simulink model "RaibertControlV10"  (R2022a)
settings: Solver=ode23t  StartTime=0.0  StopTime=10  FixedStep=1/1000  MaxStep=0.001  RelTol=1e-3  AbsTol=1e-3  EnableMultiTasking=on
values from neighbouring files (symbols this model uses):
  dphi_d_14 = 0.0    (= 0)    [initialization.m]
  dphi_d_23 = 0.0    (= 0)    [initialization.m]
  dphi_des = DesiredImpedenceValues(4)    [Controller.m]    (also in initialization.m = 0)
  dr_d_14 = 0.0    (= 0)    [initialization.m]
  dr_d_23 = 0.0    (= 0)    [initialization.m]
  dr_des = DesiredImpedenceValues(3)    [Controller.m]    (also in initialization.m = 0)
  Fpush_d_14 = 300    [initialization.m]
  Fpush_d_23 = 300    [initialization.m]
  GAIN_dx_d_14 = 0.05    [initialization.m]
  GAIN_dx_d_23 = 0.05    [initialization.m]
  Kd_phi_d_14 = 10    [initialization.m]
  Kd_phi_d_23 = 10    [initialization.m]
  Kd_r_d_14 = Kp_r_d_14*0.1    (= 60)    [initialization.m]
  Kd_r_d_23 = Kp_r_d_23*0.1    (= 50)    [initialization.m]
  Kdphi_des = DesiredImpedenceValues(8)    [Controller.m]    (also in initialization.m = 5)
  Kdr_des = DesiredImpedenceValues(6)    [Controller.m]    (also in initialization.m = 700)
  Kp_phi_d_14 = 200    [initialization.m]
  Kp_phi_d_23 = 200    [initialization.m]
  Kp_r_d_14 = 600    [initialization.m]
  Kp_r_d_23 = 500    [initialization.m]
  Kpphi_des = DesiredImpedenceValues(7)    [Controller.m]    (also in initialization.m = 50)
  Kpr_des = DesiredImpedenceValues(5)    [Controller.m]    (also in initialization.m = 700)
  phi_d_14 = 0    [initialization.m]
  phi_d_23 = 0    [initialization.m]
  phi_des = DesiredImpedenceValues(2)    [Controller.m]    (also in initialization.m = 0)
  r_d_14 = 0.38    [initialization.m]
  r_d_23 = 0.38    [initialization.m]
  r_des = DesiredImpedenceValues(1)    [Controller.m]    (also in initialization.m = 0.4)
  rthrust_d_14 = 0.3    [initialization.m]
  rthrust_d_23 = 0.3    [initialization.m]
undefined symbols (not defined in the file or in its folder): Carrier, N, Ring, T, X, Y, Z
libraries: sm_lib x136, nesl_utility x25, Multibody_Parts_Lib x4, fl_lib x4
(part 7 of 8)

== matlab function RaibertControlV10/Raibert Control14/to_dPolar ==
  data: M1_State input; dr output; dphi output; M4_State input
function [dr,dphi] = Velocity(M1_State,M4_State)
%VELOCITY
%    [DR,DPHI] = VELOCITY(THETA1,THETA2,DTHETA1,DTHETA2)

%    This function was generated by the Symbolic Math Toolbox version 8.6.
%    17-May-2022 09:32:08
theta1 = M4_State.q;
dtheta1 = M4_State.w;
theta2 = M1_State.q;
dtheta2 = M1_State.w;
dr = dtheta1.*(sin(acos(sqrt((sin(theta1-pi./2.0).*(7.0./4.0e+1)+sin(theta2+pi./2.0).*(7.0./4.0e+1)).^2+abs(cos(theta1-pi./2.0).*(7.0./4.0e+1)+cos(theta2+pi./2.0).*(7.0./4.0e+1)+3.0./2.5e+1).^2).*(5.0./3.0))+atan2(sin(theta1-pi./2.0).*(-7.0./4.0e+1)-sin(theta2+pi./2.0).*(7.0./4.0e+1),abs(cos(theta1-pi./2.0).*(7.0./4.0e+1)+cos(theta2+pi./2.0).*(7.0./4.0e+1)+3.0./2.5e+1))+6.012387278395987e-2).*(1.0./sqrt((sin(theta1-pi./2.0).*(7.0./4.0e+1)+sin(theta2+pi./2.0).*(7.0./4.0e+1)).^2+abs(cos(theta1-pi./2.0).*(7.0./4.0e+1)+cos(theta2+pi./2.0).*(7.0./4.0e+1)+3.0./2.5e+1).^2).*(cos(theta1-pi./2.0).*(sin(theta1-pi./2.0).*(7.0./4.0e+1)+sin(theta2+pi./2.0).*(7.0./4.0e+1)).*(7.0./2.0e+1)-abs(cos(theta1-pi./2.0).*(7.0./4.0e+1)+cos(theta2+pi./2.0).*(7.0./4.0e+1)+3.0./2.5e+1).*sign(cos(theta1-pi./2.0).*(7.0./4.0e+1)+cos(theta2+pi./2.0).*(7.0./4.0e+1)+3.0./2.5e+1).*sin(theta1-pi./2.0).*(7.0./2.0e+1)).*1.0./sqrt((sin(theta1-pi./2.0).*(7.0./4.0e+1)+sin(theta2+pi./2.0).*(7.0./4.0e+1)).^2.*(-2.5e+1./9.0)-abs(cos(theta1-pi./2.0).*(7.0./4.0e+1)+cos(theta2+pi./2.0).*(7.0./4.0e+1)+3.0./2.5e+1).^2.*(2.5e+1./9.0)+1.0).*(5.0./6.0)+(abs(cos(theta1-pi./2.0).*(7.0./4.0e+1)+cos(theta2+pi./2.0).*(7.0./4.0e+1)+3.0./2.5e+1).^2.*((cos(theta1-pi./2.0).*(7.0./4.0e+1))./abs(cos(theta1-pi./2.0).*(7.0./4.0e+1)+cos(theta2+pi./2.0).*(7.0./4.0e+1)+3.0./2.5e+1)+1.0./abs(cos(theta1-pi./2.0).*(7.0./4.0e+1)+cos(theta2+pi./2.0).*(7.0./4.0e+1)+3.0./2.5e+1).^2.*sign(cos(theta1-pi./2.0).*(7.0./4.0e+1)+cos(theta2+pi./2.0).*(7.0./4.0e+1)+3.0./2.5e+1).*sin(theta1-pi./2.0).*(sin(theta1-pi./2.0).*(7.0./4.0e+1)+sin(theta2+pi./2.0).*(7.0./4.0e+1)).*(7.0./4.0e+1)))./((sin(theta1-pi./2.0).*(7.0./4.0e+1)+sin(theta2+pi./2.0).*(7.0./4.0e+1)).^2+abs(cos(theta1-pi./2.0).*(7.0./4.0e+1)+cos(theta2+pi./2.0).*(7.0./4.0e+1)+3.0./2.5e+1).^2)).*(cos(acos(sqrt((sin(theta1-pi./2.0).*(7.0./4.0e+1)+sin(theta2+pi./2.0).*(7.0./4.0e+1)).^2+abs(cos(theta1-pi./2.0).*(7.0./4.0e+1)+cos(theta2+pi./2.0).*(7.0./4.0e+1)+3.0./2.5e+1).^2).*(5.0./3.0))+atan2(sin(theta1-pi./2.0).*(-7.0./4.0e+1)-sin(theta2+pi./2.0).*(7.0./4.0e+1),abs(cos(theta1-pi./2.0).*(7.0./4.0e+1)+cos(theta2+pi./2.0).*(7.0./4.0e+1)+3.0./2.5e+1))+6.012387278395987e-2).*(-3.328470665197855e-1)+cos(theta2+pi./2.0).*(7.0./4.0e+1)+3.0./5.0e+1).*6.65694133039571e-1+cos(acos(sqrt((sin(theta1-pi./2.0).*(7.0./4.0e+1)+sin(theta2+pi./2.0).*(7.0./4.0e+1)).^2+abs(cos(theta1-pi./2.0).*(7.0./4.0e+1)+cos(theta2+pi./2.0).*(7.0./4.0e+1)+3.0./2.5e+1).^2).*(5.0./3.0))+atan2(sin(theta1-pi./2.0).*(-7.0./4.0e+1)-sin(theta2+pi./2.0).*(7.0./4.0e+1),abs(cos(theta1-pi./2.0).*(7.0./4.0e+1)+cos(theta2+pi./2.0).*(7.0./4.0e+1)+3.0./2.5e+1))+6.012387278395987e-2).*(sin(acos(sqrt((sin(theta1-pi./2.0).*(7.0./4.0e+1)+sin(theta2+pi./2.0).*(7.0./4.0e+1)).^2+abs(cos(theta1-pi./2.0).*(7.0./4.0e+1)+cos(theta2+pi./2.0).*(7.0./4.0e+1)+3.0./2.5e+1).^2).*(5.0./3.0))+atan2(sin(theta1-pi./2.0).*(-7.0./4.0e+1)-sin(theta2+pi./2.0).*(7.0./4.0e+1),abs(cos(theta1-pi./2.0).*(7.0./4.0e+1)+cos(theta2+pi./2.0).*(7.0./4.0e+1)+3.0./2.5e+1))+6.012387278395987e-2).*3.328470665197855e-1+sin(theta2+pi./2.0).*(7.0./4.0e+1)).*(1.0./sqrt((sin(theta1-pi./2.0).*(7.0./4.0e+1)+sin(theta2+pi./2.0).*(7.0./4.0e+1)).^2+abs(cos(theta1-pi./2.0).*(7.0./4.0e+1)+cos(theta2+pi./2.0).*(7.0./4.0e+1)+3.0./2.5e+1).^2).*(cos(theta1-pi./2.0).*(sin(theta1-pi./2.0).*(7.0./4.0e+1)+sin(theta2+pi./2.0).*(7.0./4.0e+1)).*(7.0./2.0e+1)-abs(cos(theta1-pi./2.0).*(7.0./4.0e+1)+cos(theta2+pi./2.0).*(7.0./4.0e+1)+3.0./2.5e+1).*sign(cos(theta1-pi./2.0).*(7.0./4.0e+1)+cos(theta2+pi./2.0).*(7.0./4.0e+1)+3.0./2.5e+1).*sin(theta1-pi./2.0).*(7.0./2.0e+1)).*1.0./sqrt((sin(theta1-pi./2.0).*(7.0./4.0e+1)+sin(theta2+pi./2.0).*(7.0./4.0e+1)).^2.*(-2.5e+1./9.0)-abs(cos(theta1-pi./2.0).*(7.0./4.0e+1)+cos(theta2+pi./2.0).*(7.0./4.0e+1)+3.0./2.5e+1).^2.*(2.5e+1./9.0)+1.0).*(5.0./6.0)+(abs(cos(theta1-pi./2.0).*(7.0./4.0e+1)+cos(theta2+pi./2.0).*(7.0./4.0e+1)+3.0./2.5e+1).^2.*((cos(theta1-pi./2.0).*(7.0./4.0e+1))./abs(cos(theta1-pi./2.0).*(7.0./4.0e+1)+cos(theta2+pi./2.0).*(7.0./4.0e+1)+3.0./2.5e+1)+1.0./abs(cos(theta1-pi./2.0).*(7.0./4.0e+1)+cos(theta2+pi./2.0).*(7.0./4.0e+1)+3.0./2.5e+1).^2.*sign(cos(theta1-pi./2.0).*(7.0./4.0e+1)+cos(theta2+pi./2.0).*(7.0./4.0e+1)+3.0./2.5e+1).*sin(theta1-pi./2.0).*(sin(theta1-pi./2.0).*(7.0./4.0e+1)+sin(theta2+pi./2.0).*(7.0./4.0e+1)).*(7.0./4.0e+1)))./((sin(theta1-pi./2.0).*(7.0./4.0e+1)+sin(theta2+pi./2.0).*(7.0./4.0e+1)).^2+abs(cos(theta1-pi./2.0).*(7.0./4.0e+1)+cos(theta2+pi./2.0).*(7.0./4.0e+1)+3.0./2.5e+1).^2)).*6.65694133039571e-1).*1.0./sqrt((cos(acos(sqrt((sin(theta1-pi./2.0).*(7.0./4.0e+1)+sin(theta2+pi./2.0).*(7.0./4.0e+1)).^2+abs(cos(theta1-pi./2.0).*(7.0./4.0e+1)+cos(theta2+pi./2.0).*(7.0./4.0e+1)+3.0./2.5e+1).^2).*(5.0./3.0))+atan2(sin(theta1-pi./2.0).*(-7.0./4.0e+1)-sin(theta2+pi./2.0).*(7.0./4.0e+1),abs(cos(theta1-pi./2.0).*(7.0./4.0e+1)+cos(theta2+pi./2.0).*(7.0./4.0e+1)+3.0./2.5e+1))+6.012387278395987e-2).*(-3.328470665197855e-1)+cos(theta2+pi./2.0).*(7.0./4.0e+1)+3.0./5.0e+1).^2+(sin(acos(sqrt((sin(theta1-pi./2.0).*(7.0./4.0e+1)+sin(theta2+pi./2.0).*(7.0./4.0e+1)).^2+abs(cos(theta1-pi./2.0).*(7.0./4.0e+1)+cos(theta2+pi./2.0).*(7.0./4.0e+1)+3.0./2.5e+1).^2).*(5.0./3.0))+atan2(sin(theta1-pi./2.0).*(-7.0./4.0e+1)-sin(theta2+pi./2.0).*(7.0./4.0e+1),abs(cos(theta1-pi./2.0).*(7.0./4.0e+1)+cos(theta2+pi./2.0).*(7.0./4.0e+1)+3.0./2.5e+1))+6.012387278395987e-2).*3.328470665197855e-1+sin(theta2+pi./2.0).*(7.0./4.0e+1)).^2).*(-1.0./2.0)+(dtheta2.*((sin(acos(sqrt((sin(theta1-pi./2.0).*(7.0./4.0e+1)+sin(theta2+pi./2.0).*(7.0./4.0e+1)).^2+abs(cos(theta1-pi./2.0).*(7.0./4.0e+1)+cos(theta2+pi./2.0).*(7.0./4.0e+1)+3.0./2.5e+1).^2).*(5.0./3.0))+atan2(sin(theta1-pi./2.0).*(-7.0./4.0e+1)-sin(theta2+pi./2.0).*(7.0./4.0e+1),abs(cos(theta1-pi./2.0).*(7.0./4.0e+1)+cos(theta2+pi./2.0).*(7.0./4.0e+1)+3.0./2.5e+1))+6.012387278395987e-2).*3.328470665197855e-1+sin(theta2+pi./2.0).*(7.0./4.0e+1)).*(cos(theta2+pi./2.0).*(7.0./4.0e+1)-cos(acos(sqrt((sin(theta1-pi./2.0).*(7.0./4.0e+1)+sin(theta2+pi./2.0).*(7.0./4.0e+1)).^2+abs(cos(theta1-pi./2.0).*(7.0./4.0e+1)+cos(theta2+pi./2.0).*(7.0./4.0e+1)+3.0./2.5e+1).^2).*(5.0./3.0))+atan2(sin(theta1-pi./2.0).*(-7.0./4.0e+1)-sin(theta2+pi./2.0).*(7.0./4.0e+1),abs(cos(theta1-pi./2.0).*(7.0./4.0e+1)+cos(theta2+pi./2.0).*(7.0./4.0e+1)+3.0./2.5e+1))+6.012387278395987e-2).*(1.0./sqrt((sin(theta1-pi./2.0).*(7.0./4.0e+1)+sin(theta2+pi./2.0).*(7.0./4.0e+1)).^2+abs(cos(theta1-pi./2.0).*(7.0./4.0e+1)+cos(theta2+pi./2.0).*(7.0./4.0e+1)+3.0./2.5e+1).^2).*(cos(theta2+pi./2.0).*(sin(theta1-pi./2.0).*(7.0./4.0e+1)+sin(theta2+pi./2.0).*(7.0./4.0e+1)).*(7.0./2.0e+1)-abs(cos(theta1-pi./2.0).*(7.0./4.0e+1)+cos(theta2+pi./2.0).*(7.0./4.0e+1)+3.0./2.5e+1).*sign(cos(theta1-pi./2.0).*(7.0./4.0e+1)+cos(theta2+pi./2.0).*(7.0./4.0e+1)+3.0./2.5e+1).*sin(theta2+pi./2.0).*(7.0./2.0e+1)).*1.0./sqrt((sin(theta1-pi./2.0).*(7.0./4.0e+1)+sin(theta2+pi./2.0).*(7.0./4.0e+1)).^2.*(-2.5e+1./9.0)-abs(cos(theta1-pi./2.0).*(7.0./4.0e+1)+cos(theta2+pi./2.0).*(7.0./4.0e+1)+3.0./2.5e+1).^2.*(2.5e+1./9.0)+1.0).*(5.0./6.0)+(abs(cos(theta1-pi./2.0).*(7.0./4.0e+1)+cos(theta2+pi./2.0).*(7.0./4.0e+1)+3.0./2.5e+1).^2.*((cos(theta2+pi./2.0).*(7.0./4.0e+1))./abs(cos(theta1-pi./2.0).*(7.0./4.0e+1)+cos(theta2+pi./2.0).*(7.0./4.0e+1)+3.0./2.5e+1)+1.0./abs(cos(theta1-pi./2.0).*(7.0./4.0e+1)+cos(theta2+pi./2.0).*(7.0./4.0e+1)+3.0./2.5e+1).^2.*sign(cos(theta1-pi./2.0).*(7.0./4.0e+1)+cos(theta2+pi./2.0).*(7.0./4.0e+1)+3.0./2.5e+1).*sin(theta2+pi./2.0).*(sin(theta1-pi./2.0).*(7.0./4.0e+1)+sin(theta2+pi./2.0).*(7.0./4.0e+1)).*(7.0./4.0e+1)))./((sin(theta1-pi./2.0).*(7.0./4.0e+1)+sin(theta2+pi./2.0).*(7.0./4.0e+1)).^2+abs(cos(theta1-pi./2.0).*(7.0./4.0e+1)+cos(theta2+pi./2.0).*(7.0./4.0e+1)+3.0./2.5e+1).^2)).*3.328470665197855e-1).*2.0-(sin(theta2+pi./2.0).*(7.0./4.0e+1)+sin(acos(sqrt((sin(theta1-pi./2.0).*(7.0./4.0e+1)+sin(theta2+pi./2.0).*(7.0./4.0e+1)).^2+abs(cos(theta1-pi./2.0).*(7.0./4.0e+1)+cos(theta2+pi./2.0).*(7.0./4.0e+1)+3.0./2.5e+1).^2).*(5.0./3.0))+atan2(sin(theta1-pi./2.0).*(-7.0./4.0e+1)-sin(theta2+pi./2.0).*(7.0./4.0e+1),abs(cos(theta1-pi./2.0).*(7.0./4.0e+1)+cos(theta2+pi./2.0).*(7.0./4.0e+1)+3.0./2.5e+1))+6.012387278395987e-2).*(1.0./sqrt((sin(theta1-pi./2.0).*(7.0./4.0e+1)+sin(theta2+pi./2.0).*(7.0./4.0e+1)).^2+abs(cos(theta1-pi./2.0).*(7.0./4.0e+1)+cos(theta2+pi./2.0).*(7.0./4.0e+1)+3.0./2.5e+1).^2).*(cos(theta2+pi./2.0).*(sin(theta1-pi./2.0).*(7.0./4.0e+1)+sin(theta2+pi./2.0).*(7.0./4.0e+1)).*(7.0./2.0e+1)-abs(cos(theta1-pi./2.0).*(7.0./4.0e+1)+cos(theta2+pi./2.0).*(7.0./4.0e+1)+3.0./2.5e+1).*sign(cos(theta1-pi./2.0).*(7.0./4.0e+1)+cos(theta2+pi./2.0).*(7.0./4.0e+1)+3.0./2.5e+1).*sin(theta2+pi./2.0).*(7.0./2.0e+1)).*1.0./sqrt((sin(theta1-pi./2.0).*(7.0./4.0e+1)+sin(theta2+pi./2.0).*(7.0./4.0e+1)).^2.*(-2.5e+1./9.0)-abs(cos(theta1-pi./2.0).*(7.0./4.0e+1)+cos(theta2+pi./2.0).*(7.0./4.0e+1)+3.0./2.5e+1).^2.*(2.5e+1./9.0)+1.0).*(5.0./6.0)+(abs(cos(theta1-pi./2.0).*(7.0./4.0e+1)+cos(theta2+pi./2.0).*(7.0./4.0e+1)+3.0./2.5e+1).^2.*((cos(theta2+pi./2.0).*(7.0./4.0e+1))./abs(cos(theta1-pi./2.0).*(7.0./4.0e+1)+cos(theta2+pi./2.0).*(7.0./4.0e+1)+3.0./2.5e+1)+1.0./abs(cos(theta1-pi./2.0).*(7.0./4.0e+1)+cos(theta2+pi./2.0).*(7.0./4.0e+1)+3.0./2.5e+1).^2.*sign(cos(theta1-pi./2.0).*(7.0./4.0e+1)+cos(theta2+pi./2.0).*(7.0./4.0e+1)+3.0./2.5e+1).*sin(theta2+pi./2.0).*(sin(theta1-pi./2.0).*(7.0./4.0e+1)+sin(theta2+pi./2.0).*(7.0./4.0e+1)).*(7.0./4.0e+1)))./((sin(theta1-pi./2.0).*(7.0./4.0e+1)+sin(theta2+pi./2.0).*(7.0./4.0e+1)).^2+abs(cos(theta1-pi./2.0).*(7.0./4.0e+1)+cos(theta2+pi./2.0).*(7.0./4.0e+1)+3.0./2.5e+1).^2)).*3.328470665197855e-1).*(cos(acos(sqrt((sin(theta1-pi./2.0).*(7.0./4.0e+1)+sin(theta2+pi./2.0).*(7.0./4.0e+1)).^2+abs(cos(theta1-pi./2.0).*(7.0./4.0e+1)+cos(theta2+pi./2.0).*(7.0./4.0e+1)+3.0./2.5e+1).^2).*(5.0./3.0))+atan2(sin(theta1-pi./2.0).*(-7.0./4.0e+1)-sin(theta2+pi./2.0).*(7.0./4.0e+1),abs(cos(theta1-pi./2.0).*(7.0./4.0e+1)+cos(theta2+pi./2.0).*(7.0./4.0e+1)+3.0./2.5e+1))+6.012387278395987e-2).*(-3.328470665197855e-1)+cos(theta2+pi./2.0).*(7.0./4.0e+1)+3.0./5.0e+1).*2.0).*1.0./sqrt((cos(acos(sqrt((sin(theta1-pi./2.0).*(7.0./4.0e+1)+sin(theta2+pi./2.0).*(7.0./4.0e+1)).^2+abs(cos(theta1-pi./2.0).*(7.0./4.0e+1)+cos(theta2+pi./2.0).*(7.0./4.0e+1)+3.0./2.5e+1).^2).*(5.0./3.0))+atan2(sin(theta1-pi./2.0).*(-7.0./4.0e+1)-sin(theta2+pi./2.0).*(7.0./4.0e+1),abs(cos(theta1-pi./2.0).*(7.0./4.0e+1)+cos(theta2+pi./2.0).*(7.0./4.0e+1)+3.0./2.5e+1))+6.012387278395987e-2).*(-3.328470665197855e-1)+cos(theta2+pi./2.0).*(7.0./4.0e+1)+3.0./5.0e+1).^2+(sin(acos(sqrt((sin(theta1-pi./2.0).*(7.0./4.0e+1)+sin(theta2+pi./2.0).*(7.0./4.0e+1)).^2+abs(cos(theta1-pi./2.0).*(7.0./4.0e+1)+cos(theta2+pi./2.0).*(7.0./4.0e+1)+3.0./2.5e+1).^2).*(5.0./3.0))+atan2(sin(theta1-pi./2.0).*(-7.0./4.0e+1)-sin(theta2+pi./2.0).*(7.0./4.0e+1),abs(cos(theta1-pi./2.0).*(7.0./4.0e+1)+cos(theta2+pi./2.0).*(7.0./4.0e+1)+3.0./2.5e+1))+6.012387278395987e-2).*3.328470665197855e-1+sin(theta2+pi./2.0).*(7.0./4.0e+1)).^2))./2.0;
if nargout > 1
    dphi = (dtheta1.*((cos(acos(sqrt((sin(theta1-pi./2.0).*(7.0./4.0e+1)+sin(theta2+pi./2.0).*(7.0./4.0e+1)).^2+abs(cos(theta1-pi./2.0).*(7.0./4.0e+1)+cos(theta2+pi./2.0).*(7.0./4.0e+1)+3.0./2.5e+1).^2).*(5.0./3.0))+atan2(sin(theta1-pi./2.0).*(-7.0./4.0e+1)-sin(theta2+pi./2.0).*(7.0./4.0e+1),abs(cos(theta1-pi./2.0).*(7.0./4.0e+1)+cos(theta2+pi./2.0).*(7.0./4.0e+1)+3.0./2.5e+1))+6.012387278395987e-2).*(1.0./sqrt((sin(theta1-pi./2.0).*(7.0./4.0e+1)+sin(theta2+pi./2.0).*(7.0./4.0e+1)).^2+abs(cos(theta1-pi./2.0).*(7.0./4.0e+1)+cos(theta2+pi./2.0).*(7.0./4.0e+1)+3.0./2.5e+1).^2).*(cos(theta1-pi./2.0).*(sin(theta1-pi./2.0).*(7.0./4.0e+1)+sin(theta2+pi./2.0).*(7.0./4.0e+1)).*(7.0./2.0e+1)-abs(cos(theta1-pi./2.0).*(7.0./4.0e+1)+cos(theta2+pi./2.0).*(7.0./4.0e+1)+3.0./2.5e+1).*sign(cos(theta1-pi./2.0).*(7.0./4.0e+1)+cos(theta2+pi./2.0).*(7.0./4.0e+1)+3.0./2.5e+1).*sin(theta1-pi./2.0).*(7.0./2.0e+1)).*1.0./sqrt((sin(theta1-pi./2.0).*(7.0./4.0e+1)+sin(theta2+pi./2.0).*(7.0./4.0e+1)).^2.*(-2.5e+1./9.0)-abs(cos(theta1-pi./2.0).*(7.0./4.0e+1)+cos(theta2+pi./2.0).*(7.0./4.0e+1)+3.0./2.5e+1).^2.*(2.5e+1./9.0)+1.0).*(5.0./6.0)+(abs(cos(theta1-pi./2.0).*(7.0./4.0e+1)+cos(theta2+pi./2.0).*(7.0./4.0e+1)+3.0./2.5e+1).^2.*((cos(theta1-pi./2.0).*(7.0./4.0e+1))./abs(cos(theta1-pi./2.0).*(7.0./4.0e+1)+cos(theta2+pi./2.0).*(7.0./4.0e+1)+3.0./2.5e+1)+1.0./abs(cos(theta1-pi./2.0).*(7.0./4.0e+1)+cos(theta2+pi./2.0).*(7.0./4.0e+1)+3.0./2.5e+1).^2.*sign(cos(theta1-pi./2.0).*(7.0./4.0e+1)+cos(theta2+pi./2.0).*(7.0./4.0e+1)+3.0./2.5e+1).*sin(theta1-pi./2.0).*(sin(theta1-pi./2.0).*(7.0./4.0e+1)+sin(theta2+pi./2.0).*(7.0./4.0e+1)).*(7.0./4.0e+1)))./((sin(theta1-pi./2.0).*(7.0./4.0e+1)+sin(theta2+pi./2.0).*(7.0./4.0e+1)).^2+abs(cos(theta1-pi./2.0).*(7.0./4.0e+1)+cos(theta2+pi./2.0).*(7.0./4.0e+1)+3.0./2.5e+1).^2)).*3.328470665197855e-1)./(cos(acos(sqrt((sin(theta1-pi./2.0).*(7.0./4.0e+1)+sin(theta2+pi./2.0).*(7.0./4.0e+1)).^2+abs(cos(theta1-pi./2.0).*(7.0./4.0e+1)+cos(theta2+pi./2.0).*(7.0./4.0e+1)+3.0./2.5e+1).^2).*(5.0./3.0))+atan2(sin(theta1-pi./2.0).*(-7.0./4.0e+1)-sin(theta2+pi./2.0).*(7.0./4.0e+1),abs(cos(theta1-pi./2.0).*(7.0./4.0e+1)+cos(theta2+pi./2.0).*(7.0./4.0e+1)+3.0./2.5e+1))+6.012387278395987e-2).*(-3.328470665197855e-1)+cos(theta2+pi./2.0).*(7.0./4.0e+1)+3.0./5.0e+1)-sin(acos(sqrt((sin(theta1-pi./2.0).*(7.0./4.0e+1)+sin(theta2+pi./2.0).*(7.0./4.0e+1)).^2+abs(cos(theta1-pi./2.0).*(7.0./4.0e+1)+cos(theta2+pi./2.0).*(7.0./4.0e+1)+3.0./2.5e+1).^2).*(5.0./3.0))+atan2(sin(theta1-pi./2.0).*(-7.0./4.0e+1)-sin(theta2+pi./2.0).*(7.0./4.0e+1),abs(cos(theta1-pi./2.0).*(7.0./4.0e+1)+cos(theta2+pi./2.0).*(7.0./4.0e+1)+3.0./2.5e+1))+6.012387278395987e-2).*(sin(acos(sqrt((sin(theta1-pi./2.0).*(7.0./4.0e+1)+sin(theta2+pi./2.0).*(7.0./4.0e+1)).^2+abs(cos(theta1-pi./2.0).*(7.0./4.0e+1)+cos(theta2+pi./2.0).*(7.0./4.0e+1)+3.0./2.5e+1).^2).*(5.0./3.0))+atan2(sin(theta1-pi./2.0).*(-7.0./4.0e+1)-sin(theta2+pi./2.0).*(7.0./4.0e+1),abs(cos(theta1-pi./2.0).*(7.0./4.0e+1)+cos(theta2+pi./2.0).*(7.0./4.0e+1)+3.0./2.5e+1))+6.012387278395987e-2).*3.328470665197855e-1+sin(theta2+pi./2.0).*(7.0./4.0e+1)).*(1.0./sqrt((sin(theta1-pi./2.0).*(7.0./4.0e+1)+sin(theta2+pi./2.0).*(7.0./4.0e+1)).^2+abs(cos(theta1-pi./2.0).*(7.0./4.0e+1)+cos(theta2+pi./2.0).*(7.0./4.0e+1)+3.0./2.5e+1).^2).*(cos(theta1-pi./2.0).*(sin(theta1-pi./2.0).*(7.0./4.0e+1)+sin(theta2+pi./2.0).*(7.0./4.0e+1)).*(7.0./2.0e+1)-abs(cos(theta1-pi./2.0).*(7.0./4.0e+1)+cos(theta2+pi./2.0).*(7.0./4.0e+1)+3.0./2.5e+1).*sign(cos(theta1-pi./2.0).*(7.0./4.0e+1)+cos(theta2+pi./2.0).*(7.0./4.0e+1)+3.0./2.5e+1).*sin(theta1-pi./2.0).*(7.0./2.0e+1)).*1.0./sqrt((sin(theta1-pi./2.0).*(7.0./4.0e+1)+sin(theta2+pi./2.0).*(7.0./4.0e+1)).^2.*(-2.5e+1./9.0)-abs(cos(theta1-pi./2.0).*(7.0./4.0e+1)+cos(theta2+pi./2.0).*(7.0./4.0e+1)+3.0./2.5e+1).^2.*(2.5e+1./9.0)+1.0).*(5.0./6.0)+(abs(cos(theta1-pi./2.0).*(7.0./4.0e+1)+cos(theta2+pi./2.0).*(7.0./4.0e+1)+3.0./2.5e+1).^2.*((cos(theta1-pi./2.0).*(7.0./4.0e+1))./abs(cos(theta1-pi./2.0).*(7.0./4.0e+1)+cos(theta2+pi./2.0).*(7.0./4.0e+1)+3.0./2.5e+1)+1.0./abs(cos(theta1-pi./2.0).*(7.0./4.0e+1)+cos(theta2+pi./2.0).*(7.0./4.0e+1)+3.0./2.5e+1).^2.*sign(cos(theta1-pi./2.0).*(7.0./4.0e+1)+cos(theta2+pi./2.0).*(7.0./4.0e+1)+3.0./2.5e+1).*sin(theta1-pi./2.0).*(sin(theta1-pi./2.0).*(7.0./4.0e+1)+sin(theta2+pi./2.0).*(7.0./4.0e+1)).*(7.0./4.0e+1)))./((sin(theta1-pi./2.0).*(7.0./4.0e+1)+sin(theta2+pi./2.0).*(7.0./4.0e+1)).^2+abs(cos(theta1-pi./2.0).*(7.0./4.0e+1)+cos(theta2+pi./2.0).*(7.0./4.0e+1)+3.0./2.5e+1).^2)).*1.0./(cos(acos(sqrt((sin(theta1-pi./2.0).*(7.0./4.0e+1)+sin(theta2+pi./2.0).*(7.0./4.0e+1)).^2+abs(cos(theta1-pi./2.0).*(7.0./4.0e+1)+cos(theta2+pi./2.0).*(7.0./4.0e+1)+3.0./2.5e+1).^2).*(5.0./3.0))+atan2(sin(theta1-pi./2.0).*(-7.0./4.0e+1)-sin(theta2+pi./2.0).*(7.0./4.0e+1),abs(cos(theta1-pi./2.0).*(7.0./4.0e+1)+cos(theta2+pi./2.0).*(7.0./4.0e+1)+3.0./2.5e+1))+6.012387278395987e-2).*(-3.328470665197855e-1)+cos(theta2+pi./2.0).*(7.0./4.0e+1)+3.0./5.0e+1).^2.*3.328470665197855e-1).*(cos(acos(sqrt((sin(theta1-pi./2.0).*(7.0./4.0e+1)+sin(theta2+pi./2.0).*(7.0./4.0e+1)).^2+abs(cos(theta1-pi./2.0).*(7.0./4.0e+1)+cos(theta2+pi./2.0).*(7.0./4.0e+1)+3.0./2.5e+1).^2).*(5.0./3.0))+atan2(sin(theta1-pi./2.0).*(-7.0./4.0e+1)-sin(theta2+pi./2.0).*(7.0./4.0e+1),abs(cos(theta1-pi./2.0).*(7.0./4.0e+1)+cos(theta2+pi./2.0).*(7.0./4.0e+1)+3.0./2.5e+1))+6.012387278395987e-2).*(-3.328470665197855e-1)+cos(theta2+pi./2.0).*(7.0./4.0e+1)+3.0./5.0e+1).^2)./((cos(acos(sqrt((sin(theta1-pi./2.0).*(7.0./4.0e+1)+sin(theta2+pi./2.0).*(7.0./4.0e+1)).^2+abs(cos(theta1-pi./2.0).*(7.0./4.0e+1)+cos(theta2+pi./2.0).*(7.0./4.0e+1)+3.0./2.5e+1).^2).*(5.0./3.0))+atan2(sin(theta1-pi./2.0).*(-7.0./4.0e+1)-sin(theta2+pi./2.0).*(7.0./4.0e+1),abs(cos(theta1-pi./2.0).*(7.0./4.0e+1)+cos(theta2+pi./2.0).*(7.0./4.0e+1)+3.0./2.5e+1))+6.012387278395987e-2).*(-3.328470665197855e-1)+cos(theta2+pi./2.0).*(7.0./4.0e+1)+3.0./5.0e+1).^2+(sin(acos(sqrt((sin(theta1-pi./2.0).*(7.0./4.0e+1)+sin(theta2+pi./2.0).*(7.0./4.0e+1)).^2+abs(cos(theta1-pi./2.0).*(7.0./4.0e+1)+cos(theta2+pi./2.0).*(7.0./4.0e+1)+3.0./2.5e+1).^2).*(5.0./3.0))+atan2(sin(theta1-pi./2.0).*(-7.0./4.0e+1)-sin(theta2+pi./2.0).*(7.0./4.0e+1),abs(cos(theta1-pi./2.0).*(7.0./4.0e+1)+cos(theta2+pi./2.0).*(7.0./4.0e+1)+3.0./2.5e+1))+6.012387278395987e-2).*3.328470665197855e-1+sin(theta2+pi./2.0).*(7.0./4.0e+1)).^2)-(dtheta2.*((cos(theta2+pi./2.0).*(7.0./4.0e+1)-cos(acos(sqrt((sin(theta1-pi./2.0).*(7.0./4.0e+1)+sin(theta2+pi./2.0).*(7.0./4.0e+1)).^2+abs(cos(theta1-pi./2.0).*(7.0./4.0e+1)+cos(theta2+pi./2.0).*(7.0./4.0e+1)+3.0./2.5e+1).^2).*(5.0./3.0))+atan2(sin(theta1-pi./2.0).*(-7.0./4.0e+1)-sin(theta2+pi./2.0).*(7.0./4.0e+1),abs(cos(theta1-pi./2.0).*(7.0./4.0e+1)+cos(theta2+pi./2.0).*(7.0./4.0e+1)+3.0./2.5e+1))+6.012387278395987e-2).*(1.0./sqrt((sin(theta1-pi./2.0).*(7.0./4.0e+1)+sin(theta2+pi./2.0).*(7.0./4.0e+1)).^2+abs(cos(theta1-pi./2.0).*(7.0./4.0e+1)+cos(theta2+pi./2.0).*(7.0./4.0e+1)+3.0./2.5e+1).^2).*(cos(theta2+pi./2.0).*(sin(theta1-pi./2.0).*(7.0./4.0e+1)+sin(theta2+pi./2.0).*(7.0./4.0e+1)).*(7.0./2.0e+1)-abs(cos(theta1-pi./2.0).*(7.0./4.0e+1)+cos(theta2+pi./2.0).*(7.0./4.0e+1)+3.0./2.5e+1).*sign(cos(theta1-pi./2.0).*(7.0./4.0e+1)+cos(theta2+pi./2.0).*(7.0./4.0e+1)+3.0./2.5e+1).*sin(theta2+pi./2.0).*(7.0./2.0e+1)).*1.0./sqrt((sin(theta1-pi./2.0).*(7.0./4.0e+1)+sin(theta2+pi./2.0).*(7.0./4.0e+1)).^2.*(-2.5e+1./9.0)-abs(cos(theta1-pi./2.0).*(7.0./4.0e+1)+cos(theta2+pi./2.0).*(7.0./4.0e+1)+3.0./2.5e+1).^2.*(2.5e+1./9.0)+1.0).*(5.0./6.0)+(abs(cos(theta1-pi./2.0).*(7.0./4.0e+1)+cos(theta2+pi./2.0).*(7.0./4.0e+1)+3.0./2.5e+1).^2.*((cos(theta2+pi./2.0).*(7.0./4.0e+1))./abs(cos(theta1-pi./2.0).*(7.0./4.0e+1)+cos(theta2+pi./2.0).*(7.0./4.0e+1)+3.0./2.5e+1)+1.0./abs(cos(theta1-pi./2.0).*(7.0./4.0e+1)+cos(theta2+pi./2.0).*(7.0./4.0e+1)+3.0./2.5e+1).^2.*sign(cos(theta1-pi./2.0).*(7.0./4.0e+1)+cos(theta2+pi./2.0).*(7.0./4.0e+1)+3.0./2.5e+1).*sin(theta2+pi./2.0).*(sin(theta1-pi./2.0).*(7.0./4.0e+1)+sin(theta2+pi./2.0).*(7.0./4.0e+1)).*(7.0./4.0e+1)))./((sin(theta1-pi./2.0).*(7.0./4.0e+1)+sin(theta2+pi./2.0).*(7.0./4.0e+1)).^2+abs(cos(theta1-pi./2.0).*(7.0./4.0e+1)+cos(theta2+pi./2.0).*(7.0./4.0e+1)+3.0./2.5e+1).^2)).*3.328470665197855e-1)./(cos(acos(sqrt((sin(theta1-pi./2.0).*(7.0./4.0e+1)+sin(theta2+pi./2.0).*(7.0./4.0e+1)).^2+abs(cos(theta1-pi./2.0).*(7.0./4.0e+1)+cos(theta2+pi./2.0).*(7.0./4.0e+1)+3.0./2.5e+1).^2).*(5.0./3.0))+atan2(sin(theta1-pi./2.0).*(-7.0./4.0e+1)-sin(theta2+pi./2.0).*(7.0./4.0e+1),abs(cos(theta1-pi./2.0).*(7.0./4.0e+1)+cos(theta2+pi./2.0).*(7.0./4.0e+1)+3.0./2.5e+1))+6.012387278395987e-2).*(-3.328470665197855e-1)+cos(theta2+pi./2.0).*(7.0./4.0e+1)+3.0./5.0e+1)+(sin(acos(sqrt((sin(theta1-pi./2.0).*(7.0./4.0e+1)+sin(theta2+pi./2.0).*(7.0./4.0e+1)).^2+abs(cos(theta1-pi./2.0).*(7.0./4.0e+1)+cos(theta2+pi./2.0).*(7.0./4.0e+1)+3.0./2.5e+1).^2).*(5.0./3.0))+atan2(sin(theta1-pi./2.0).*(-7.0./4.0e+1)-sin(theta2+pi./2.0).*(7.0./4.0e+1),abs(cos(theta1-pi./2.0).*(7.0./4.0e+1)+cos(theta2+pi./2.0).*(7.0./4.0e+1)+3.0./2.5e+1))+6.012387278395987e-2).*3.328470665197855e-1+sin(theta2+pi./2.0).*(7.0./4.0e+1)).*(sin(theta2+pi./2.0).*(7.0./4.0e+1)+sin(acos(sqrt((sin(theta1-pi./2.0).*(7.0./4.0e+1)+sin(theta2+pi./2.0).*(7.0./4.0e+1)).^2+abs(cos(theta1-pi./2.0).*(7.0./4.0e+1)+cos(theta2+pi./2.0).*(7.0./4.0e+1)+3.0./2.5e+1).^2).*(5.0./3.0))+atan2(sin(theta1-pi./2.0).*(-7.0./4.0e+1)-sin(theta2+pi./2.0).*(7.0./4.0e+1),abs(cos(theta1-pi./2.0).*(7.0./4.0e+1)+cos(theta2+pi./2.0).*(7.0./4.0e+1)+3.0./2.5e+1))+6.012387278395987e-2).*(1.0./sqrt((sin(theta1-pi./2.0).*(7.0./4.0e+1)+sin(theta2+pi./2.0).*(7.0./4.0e+1)).^2+abs(cos(theta1-pi./2.0).*(7.0./4.0e+1)+cos(theta2+pi./2.0).*(7.0./4.0e+1)+3.0./2.5e+1).^2).*(cos(theta2+pi./2.0).*(sin(theta1-pi./2.0).*(7.0./4.0e+1)+sin(theta2+pi./2.0).*(7.0./4.0e+1)).*(7.0./2.0e+1)-abs(cos(theta1-pi./2.0).*(7.0./4.0e+1)+cos(theta2+pi./2.0).*(7.0./4.0e+1)+3.0./2.5e+1).*sign(cos(theta1-pi./2.0).*(7.0./4.0e+1)+cos(theta2+pi./2.0).*(7.0./4.0e+1)+3.0./2.5e+1).*sin(theta2+pi./2.0).*(7.0./2.0e+1)).*1.0./sqrt((sin(theta1-pi./2.0).*(7.0./4.0e+1)+sin(theta2+pi./2.0).*(7.0./4.0e+1)).^2.*(-2.5e+1./9.0)-abs(cos(theta1-pi./2.0).*(7.0./4.0e+1)+cos(theta2+pi./2.0).*(7.0./4.0e+1)+3.0./2.5e+1).^2.*(2.5e+1./9.0)+1.0).*(5.0./6.0)+(abs(cos(theta1-pi./2.0).*(7.0./4.0e+1)+cos(theta2+pi./2.0).*(7.0./4.0e+1)+3.0./2.5e+1).^2.*((cos(theta2+pi./2.0).*(7.0./4.0e+1))./abs(cos(theta1-pi./2.0).*(7.0./4.0e+1)+cos(theta2+pi./2.0).*(7.0./4.0e+1)+3.0./2.5e+1)+1.0./abs(cos(theta1-pi./2.0).*(7.0./4.0e+1)+cos(theta2+pi./2.0).*(7.0./4.0e+1)+3.0./2.5e+1).^2.*sign(cos(theta1-pi./2.0).*(7.0./4.0e+1)+cos(theta2+pi./2.0).*(7.0./4.0e+1)+3.0./2.5e+1).*sin(theta2+pi./2.0).*(sin(theta1-pi./2.0).*(7.0./4.0e+1)+sin(theta2+pi./2.0).*(7.0./4.0e+1)).*(7.0./4.0e+1)))./((sin(theta1-pi./2.0).*(7.0./4.0e+1)+sin(theta2+pi./2.0).*(7.0./4.0e+1)).^2+abs(cos(theta1-pi./2.0).*(7.0./4.0e+1)+cos(theta2+pi./2.0).*(7.0./4.0e+1)+3.0./2.5e+1).^2)).*3.328470665197855e-1).*1.0./(cos(acos(sqrt((sin(theta1-pi./2.0).*(7.0./4.0e+1)+sin(theta2+pi./2.0).*(7.0./4.0e+1)).^2+abs(cos(theta1-pi./2.0).*(7.0./4.0e+1)+cos(theta2+pi./2.0).*(7.0./4.0e+1)+3.0./2.5e+1).^2).*(5.0./3.0))+atan2(sin(theta1-pi./2.0).*(-7.0./4.0e+1)-sin(theta2+pi./2.0).*(7.0./4.0e+1),abs(cos(theta1-pi./2.0).*(7.0./4.0e+1)+cos(theta2+pi./2.0).*(7.0./4.0e+1)+3.0./2.5e+1))+6.012387278395987e-2).*(-3.328470665197855e-1)+cos(theta2+pi./2.0).*(7.0./4.0e+1)+3.0./5.0e+1).^2).*(cos(acos(sqrt((sin(theta1-pi./2.0).*(7.0./4.0e+1)+sin(theta2+pi./2.0).*(7.0./4.0e+1)).^2+abs(cos(theta1-pi./2.0).*(7.0./4.0e+1)+cos(theta2+pi./2.0).*(7.0./4.0e+1)+3.0./2.5e+1).^2).*(5.0./3.0))+atan2(sin(theta1-pi./2.0).*(-7.0./4.0e+1)-sin(theta2+pi./2.0).*(7.0./4.0e+1),abs(cos(theta1-pi./2.0).*(7.0./4.0e+1)+cos(theta2+pi./2.0).*(7.0./4.0e+1)+3.0./2.5e+1))+6.012387278395987e-2).*(-3.328470665197855e-1)+cos(theta2+pi./2.0).*(7.0./4.0e+1)+3.0./5.0e+1).^2)./((cos(acos(sqrt((sin(theta1-pi./2.0).*(7.0./4.0e+1)+sin(theta2+pi./2.0).*(7.0./4.0e+1)).^2+abs(cos(theta1-pi./2.0).*(7.0./4.0e+1)+cos(theta2+pi./2.0).*(7.0./4.0e+1)+3.0./2.5e+1).^2).*(5.0./3.0))+atan2(sin(theta1-pi./2.0).*(-7.0./4.0e+1)-sin(theta2+pi./2.0).*(7.0./4.0e+1),abs(cos(theta1-pi./2.0).*(7.0./4.0e+1)+cos(theta2+pi./2.0).*(7.0./4.0e+1)+3.0./2.5e+1))+6.012387278395987e-2).*(-3.328470665197855e-1)+cos(theta2+pi./2.0).*(7.0./4.0e+1)+3.0./5.0e+1).^2+(sin(acos(sqrt((sin(theta1-pi./2.0).*(7.0./4.0e+1)+sin(theta2+pi./2.0).*(7.0./4.0e+1)).^2+abs(cos(theta1-pi./2.0).*(7.0./4.0e+1)+cos(theta2+pi./2.0).*(7.0./4.0e+1)+3.0./2.5e+1).^2).*(5.0./3.0))+atan2(sin(theta1-pi./2.0).*(-7.0./4.0e+1)-sin(theta2+pi./2.0).*(7.0./4.0e+1),abs(cos(theta1-pi./2.0).*(7.0./4.0e+1)+cos(theta2+pi./2.0).*(7.0./4.0e+1)+3.0./2.5e+1))+6.012387278395987e-2).*3.328470665197855e-1+sin(theta2+pi./2.0).*(7.0./4.0e+1)).^2);
end

== matlab function RaibertControlV10/Raibert Control M23/MATLAB Function ==
  data: M2_State input; JT11 output; M3_State input; JT12 output; JT21 output; JT22 output
function [JT11,JT12,JT21,JT22] = Jacobian_Transpose(M2_State,M3_State)
%JACOBIAN_TRANSPOSE
%    [JT11,JT12,JT21,JT22] = JACOBIAN_TRANSPOSE(THETA1,THETA2)

%    This function was generated by the Symbolic Math Toolbox version 8.6.
%    17-May-2022 09:32:09
theta1 = -M3_State.q;
theta2 = -M2_State.q;

t2 = pi./2.0;
t3 = -t2;
t4 = t2+theta2;
t5 = t3+theta1;
t6 = cos(t4);
t7 = sin(t4);
t8 = cos(t5);
t9 = sin(t5);
t10 = t6.*(7.0./4.0e+1);
t11 = t7.*(7.0./4.0e+1);
t14 = t7.*1.75e-1i;
t12 = t8.*(7.0./4.0e+1);
t13 = t9.*(7.0./4.0e+1);
t15 = t9.*1.75e-1i;
t16 = -t14;
t17 = -t15;
t18 = t11+t13;
t20 = t10+t12+3.0./2.5e+1;
t19 = t18.^2;
t21 = abs(t20);
t22 = sign(t20);
t29 = t6.*t18.*(7.0./2.0e+1);
t31 = t8.*t18.*(7.0./2.0e+1);
t23 = t21.^2;
t24 = 1.0./t21;
t26 = t19.*(2.5e+1./9.0);
t35 = t16+t17+t21;
t42 = t7.*t21.*t22.*(7.0./2.0e+1);
t43 = t9.*t21.*t22.*(7.0./2.0e+1);
t25 = 1.0./t23;
t27 = -t26;
t28 = t23.*(2.5e+1./9.0);
t32 = t10.*t24;
t33 = t12.*t24;
t34 = t19+t23;
t36 = angle(t35);
t44 = -t42;
t45 = -t43;
t30 = -t28;
t37 = 1.0./t34;
t38 = sqrt(t34);
t48 = t11.*t18.*t22.*t25;
t49 = t13.*t18.*t22.*t25;
t50 = t29+t44;
t51 = t31+t45;
t39 = 1.0./t38;
t40 = t38.*(5.0./3.0);
t46 = t27+t30+1.0;
t52 = t32+t48;
t53 = t33+t49;
t41 = acos(t40);
t47 = 1.0./sqrt(t46);
t66 = t23.*t37.*t52;
t67 = t23.*t37.*t53;
t54 = t36+t41+6.012387278395987e-2;
t68 = t39.*t47.*t50.*(5.0./6.0);
t69 = t39.*t47.*t51.*(5.0./6.0);
t55 = cos(t54);
t56 = sin(t54);
t73 = t66+t68;
t74 = t67+t69;
t57 = t55.*3.328470665197855e-1;
t58 = t56.*3.328470665197855e-1;
t77 = t55.*t73.*(-3.328470665197855e-1);
t59 = -t57;
t60 = t11+t58;
t75 = t57.*t73;
t76 = t58.*t73;
t79 = t10+t77;
t61 = t60.^2;
t62 = t10+t59+3.0./5.0e+1;
t78 = t11+t76;
t63 = t62.^2;
t64 = 1.0./t62;
t65 = 1.0./t63;
t70 = t61+t63;
t71 = 1.0./t70;
t72 = 1.0./sqrt(t70);
JT11 = t72.*(t55.*t60.*t74.*6.65694133039571e-1+t56.*t62.*t74.*6.65694133039571e-1).*(-1.0./2.0);
if nargout > 1
    JT12 = t63.*t71.*(t57.*t64.*t74-t56.*t60.*t65.*t74.*3.328470665197855e-1);
end
if nargout > 2
    JT21 = (t72.*(t60.*t79.*2.0-t62.*t78.*2.0))./2.0;
end
if nargout > 3
    JT22 = -t63.*t71.*(t64.*t79+t60.*t65.*t78);
end

== matlab function RaibertControlV10/Raibert Control M23/MATLAB Function3 ==
  settings: updateMethod=DISCRETE
  data: startButton input; bodyState input; DesiredImpedenceValues input; DesiredRaibertValues input; tau1 output; PolarState input; JacobianValues input; tau2 output; ctrl_state output; Kd output
function [tau1,tau2,ctrl_state,Kd]  = RController(startButton,bodyState,DesiredImpedenceValues,DesiredRaibertValues,PolarState,JacobianValues)
   [B, ctrl_state] =  Controller(startButton,bodyState,DesiredImpedenceValues,DesiredRaibertValues,PolarState,JacobianValues);
   tau1 = -B(1);
   tau2 = -B(2);
   if ctrl_state == State.Thrust
       Kd = 0;
   else
       Kd = 0;
   end
end

== matlab function RaibertControlV10/Raibert Control M23/to_Polar ==
  data: M2_State input; r output; phi output; M3_State input
function [r,phi] = Position(M2_State,M3_State)
%POSITION
%    [R,PHI] = POSITION(THETA1,THETA2)

%    This function was generated by the Symbolic Math Toolbox version 8.6.
%    17-May-2022 09:32:07

theta1 = -M3_State.q;
theta2 = -M2_State.q;

r = sqrt((cos(acos(sqrt((sin(theta1-pi./2.0).*(7.0./4.0e+1)+sin(theta2+pi./2.0).*(7.0./4.0e+1)).^2+abs(cos(theta1-pi./2.0).*(7.0./4.0e+1)+cos(theta2+pi./2.0).*(7.0./4.0e+1)+3.0./2.5e+1).^2).*(5.0./3.0))+atan2(sin(theta1-pi./2.0).*(-7.0./4.0e+1)-sin(theta2+pi./2.0).*(7.0./4.0e+1),abs(cos(theta1-pi./2.0).*(7.0./4.0e+1)+cos(theta2+pi./2.0).*(7.0./4.0e+1)+3.0./2.5e+1))+6.012387278395987e-2).*(-3.328470665197855e-1)+cos(theta2+pi./2.0).*(7.0./4.0e+1)+3.0./5.0e+1).^2+(sin(acos(sqrt((sin(theta1-pi./2.0).*(7.0./4.0e+1)+sin(theta2+pi./2.0).*(7.0./4.0e+1)).^2+abs(cos(theta1-pi./2.0).*(7.0./4.0e+1)+cos(theta2+pi./2.0).*(7.0./4.0e+1)+3.0./2.5e+1).^2).*(5.0./3.0))+atan2(sin(theta1-pi./2.0).*(-7.0./4.0e+1)-sin(theta2+pi./2.0).*(7.0./4.0e+1),abs(cos(theta1-pi./2.0).*(7.0./4.0e+1)+cos(theta2+pi./2.0).*(7.0./4.0e+1)+3.0./2.5e+1))+6.012387278395987e-2).*3.328470665197855e-1+sin(theta2+pi./2.0).*(7.0./4.0e+1)).^2);
if nargout > 1
    phi = pi./2.0-angle(cos(acos(sqrt((sin(theta1-pi./2.0).*(7.0./4.0e+1)+sin(theta2+pi./2.0).*(7.0./4.0e+1)).^2+abs(cos(theta1-pi./2.0).*(7.0./4.0e+1)+cos(theta2+pi./2.0).*(7.0./4.0e+1)+3.0./2.5e+1).^2).*(5.0./3.0))+atan2(sin(theta1-pi./2.0).*(-7.0./4.0e+1)-sin(theta2+pi./2.0).*(7.0./4.0e+1),abs(cos(theta1-pi./2.0).*(7.0./4.0e+1)+cos(theta2+pi./2.0).*(7.0./4.0e+1)+3.0./2.5e+1))+6.012387278395987e-2).*(-3.328470665197855e-1)+sin(acos(sqrt((sin(theta1-pi./2.0).*(7.0./4.0e+1)+sin(theta2+pi./2.0).*(7.0./4.0e+1)).^2+abs(cos(theta1-pi./2.0).*(7.0./4.0e+1)+cos(theta2+pi./2.0).*(7.0./4.0e+1)+3.0./2.5e+1).^2).*(5.0./3.0))+atan2(sin(theta1-pi./2.0).*(-7.0./4.0e+1)-sin(theta2+pi./2.0).*(7.0./4.0e+1),abs(cos(theta1-pi./2.0).*(7.0./4.0e+1)+cos(theta2+pi./2.0).*(7.0./4.0e+1)+3.0./2.5e+1))+6.012387278395987e-2).*3.328470665197855e-1i+cos(theta2+pi./2.0).*(7.0./4.0e+1)+sin(theta2+pi./2.0).*1.75e-1i+3.0./5.0e+1);
end
